simulink model "rpendtemplate"  (R2018a)
settings: Solver=ode45  StartTime=0.0  StopTime=15  RelTol=1e-3  EnableMultiTasking=on
InitFcn:
  | initLinSysID
values from neighbouring files (symbols this model uses):
  Ae = [A B*Ct; zeros(2,4) At]    [initLinSysID.m]    (also in linControl.m)
  Be = [zeros(4,1);Bt]    [initLinSysID.m]    (also in linControl.m)
  Ce = [1 0 0 0 0 0 ... (first row only)    [initLinSysID.m]    (also in linControl.m)
  h = 0.01    [LinSysID.m]    (also in initLinSysID.m = 0.005)
  K = sys.K    [LinSysID.m]
  L = place(Ae',Ce',obsp)    [initLinSysID.m]    (also in linControl.m)
  x0 = zeros(nx,1)    [LinSysID.m]    (also in initLinSysID.m = [0.49*pi 0.49*pi 0 0])
libraries: simulink x2
settings Model: Creator=rbabuska  LastModifiedBy=geert
settings DataIOCC: LimitDataPoints=on  SaveFormat=Array  SignalLoggingName=sigsOut
settings OptimizationCC: BooleanDataType=off  ExpressionDepthLimit=2147483647  InitFltsAndDblsToZero=on  LifeSpan=inf
settings DebuggingCC: SaveWithParameterizedLinksMsg=none  SignalResolutionControl=TryResolveAllWithWarning  MultiTaskDSMMsg=warning  MultiTaskCondExecSysMsg=none  AllowSymbolicDim=off  StateNameClashWarn=warning  SFUnexpectedBacktrackingDiag=warning  SFNoUnconditionalDefaultTransitionDiag=warning  SFExecutionAtInitializationDiag=none
settings HardwareCC: ProdBitPerPointer=32  ProdBitPerSizeT=32  ProdBitPerPtrDiffT=32  ProdLargestAtomicFloat=None  ProdIntDivRoundTo=Undefined  ProdEndianess=Unspecified  ProdWordSize=32  ProdHWDeviceType=32-bit Generic  TargetUnknown=on
settings ModelReferenceCC: PropagateSignalLabelsOutOfModel=off
settings CodeAppCC: StateflowObjectComments=on
settings GRTTargetCC: TargetFcnLib=ansi_tfl_tmw.mat  TargetLangStandard=C89/C90 (ANSI)  GeneratePreprocessorConditionals=Disable all  CombineOutputUpdateFcns=off  GRTInterface=on
settings ConfigComp: CovMetricSettings=dw  CovHtmlReporting=on  CovSaveCumulativeToWorkspaceVar=on  CovSaveSingleToWorkspaceVar=on  CovExternalEMLEnable=off

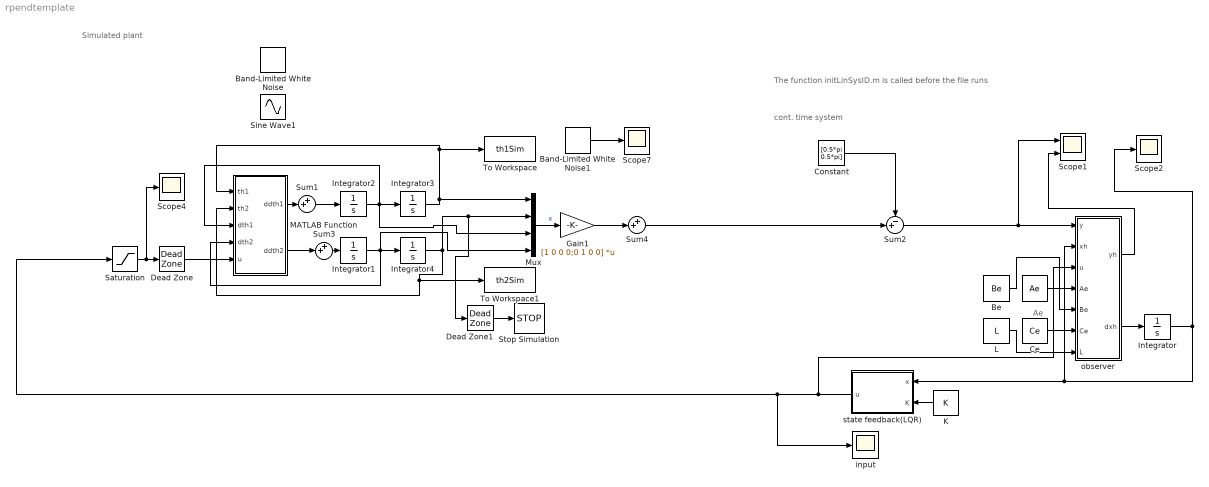
== system rpendtemplate ==
  note: cont. time system
  note: Ae
  note: The function initLinSysID.m is called before the file runs
  note: Simulated plant
  " " : Constant  Value=Ae
  Band-Limited White Noise : simulink/Sources/Band-Limited White Noise  Cov=[0]  Ts=h  seed=[23355]
  Band-Limited White Noise1 : simulink/Sources/Band-Limited White Noise  Cov=[0.0001]  Ts=h  seed=[254345]
  Be : Constant  Value=Be
  "Ce " : Constant  Value=Ce
  Constant : Constant  Value=[0.5*pi 0.5*pi]
  Dead Zone : DeadZone  LowerValue=-0.3  UpperValue=0.3  SaturateOnIntegerOverflow=on
  Dead Zone1 : DeadZone  LowerValue=0  UpperValue=pi  SaturateOnIntegerOverflow=on
  Gain1 : Gain  Gain=[1 0 0 0;0 1 0 0]  Multiplication=Matrix(K*u)
  Integrator : Integrator  InitialCondition=[0;0;0;0;0;0]
  Integrator1 : Integrator  InitialCondition=x0(4)
  Integrator2 : Integrator  InitialCondition=x0(3)
  Integrator3 : Integrator  InitialCondition=x0(1)  WrapState=on
  Integrator4 : Integrator  InitialCondition=x0(2)  WrapState=on
  "K " : Constant  Value=K
  L : Constant  Value=L
  MATLAB Function : MATLAB Function  TreatAsAtomicUnit=on
  Mux : Mux
  Saturation : Saturate  UpperLimit=1  LowerLimit=-1
  Scope1 : Scope  NumInputPorts=2
  Scope2 : Scope
  Scope4 : Scope
  Scope7 : Scope
  Sine Wave1 : Sin  Amplitude=0  Frequency=10  SampleTime=0
  Stop Simulation : Stop
  Sum1 : Sum  Inputs=++|
  Sum2 : Sum  Inputs=-+|
  Sum3 : Sum  Inputs=++|
  Sum4 : Sum  Inputs=++|
  To Workspace : ToWorkspace  VariableName=th1Sim  SampleTime=-1
  To Workspace1 : ToWorkspace  VariableName=th2Sim  SampleTime=-1
  "input " : Scope
  observer : MATLAB Function  TreatAsAtomicUnit=on
  state feedback(LQR) : MATLAB Function  TreatAsAtomicUnit=on
  wires:
  observer/2(dxh) -> Integrator/1
  Integrator/1 -> observer/2(xh), state feedback(LQR)/1(x), Scope2/1
  state feedback(LQR)/1(u) -> observer/3(u), Saturation/1, "input "/1
  observer/1(yh) -> Scope1/2
  "K "/1 -> state feedback(LQR)/2(K)
  " "/1 -> observer/4(Ae)
  Be/1 -> observer/5(Be)
  "Ce "/1 -> observer/6(Ce)
  L/1 -> observer/7(L)
  MATLAB Function/2(ddth2) -> Sum3/2
  Dead Zone/1 -> MATLAB Function/5(u)
  Saturation/1 -> Scope4/1, Dead Zone/1
  Sum1/1 -> Integrator2/1
  MATLAB Function/1(ddth1) -> Sum1/2
  Dead Zone1/1 -> Stop Simulation/1
  Integrator2/1 -> Mux/3, MATLAB Function/3(dth1), Integrator3/1
  Integrator1/1 -> Mux/4, MATLAB Function/4(dth2), Integrator4/1
  Sum3/1 -> Integrator1/1
  Integrator3/1 -> MATLAB Function/1(th1), To Workspace/1, Mux/1
  Mux/1 -> Gain1/1  "x"
  Integrator4/1 -> MATLAB Function/2(th2), To Workspace1/1, Mux/2, Dead Zone1/1
  Band-Limited White Noise1/1 -> Scope7/1
  Gain1/1 -> Sum4/2
  Sum2/1 -> Scope1/1, observer/1(y)
  Sum4/1 -> Sum2/2
  Constant/1 -> Sum2/1

== matlab function rpendtemplate/state feedback(LQR) ==
  data: x input; u output; K input
function u = K(x,K)
u = -K'*x;

== matlab function rpendtemplate/observer ==
  data: yh output; y input; dxh output; xh input; u input; Ae input; Be input; Ce input; L input
function [yh,dxh] = obs(y,xh,u,Ae,Be,Ce,L)
yh = Ce*xh;
dxh = Ae*xh+Be*u+L'*(y-yh);

== matlab function rpendtemplate/MATLAB Function ==
  data: th1 input; ddth1 output; th2 input; dth1 input; dth2 input; ddth2 output; u input
function [ddth1,ddth2] = pendubot(th1,th2,dth1,dth2,u)
%INPUT
% time(t), x(th1,th2,dth1,dth2)
%OUTPUT
% second time-derivative of theta_1(ddth1) and theta_2(ddth2)

% Set params
l1 = 0.1;
g = 9.806; 

m1 = 0.18;
m2 = 0.06;

c1 = 0.06;
c2 = 0.0628;
J1 = 0.037;
J2 = 0.00011; 

K = 1.8;
k1 = 0.35;
k2 = 0.0002;

% Set equ's
g11 = m1*c1^2+m2*l1^2+J1;
g21 = m2*l1*c2*cos(th1-th2);
g12 = m2*l1*c2*cos(th1-th2);
g22 = m2*c2^2+J2;
detG = g11*g22-g21*g12; 

V1 = g*cos(th1)*(m1*c1+m2*l1);
V2 = g*c2*m2*cos(th2);
gradV1 = (1/detG)*(g22*V1-g12*V2);
gradV2 = (1/detG)*(g11*V2-g21*V1);

Fth11 = -(1/detG)*g22*(k1*dth1);
Fth12 = (1/detG)*g21*(k1*dth1); 
Fth21 = (1/detG)*g21*k2*dth2;
Fth22 = -(1/detG)*g11*k2*dth2; 
Gam111 = (1/detG)*(0.5*m2^2*l1^2*c2^2*sin(2*(th1-th2)));
Gam122 = -(1/detG)*g22*(m2*l1*c2*sin(th1-th2)); 
Gam211 = (1/detG)*g11*(m2*l1*c2*sin(th1-th2));
Gam222 = -(1/detG)*(0.5*m2^2*l1^2*c2^2*sin(2*(th1-th2)));


Fu1 = 1/detG*g22*K*u;
Fu2 = -1/detG*g12*K*u; 

ddth1 = Fth11+Fth21-Gam111*dth1^2-Gam122*dth2^2+Fu1-gradV1;
ddth2 = Fth12+Fth22-Gam211*dth1^2-Gam222*dth2^2+Fu2-gradV2;
